simulink model "simulation"  (R2017b)
settings: Solver=VariableStepAuto  StartTime=0.0  StopTime=10.0  RelTol=1e-3
settings Model: Creator=max  LastModifiedBy=max

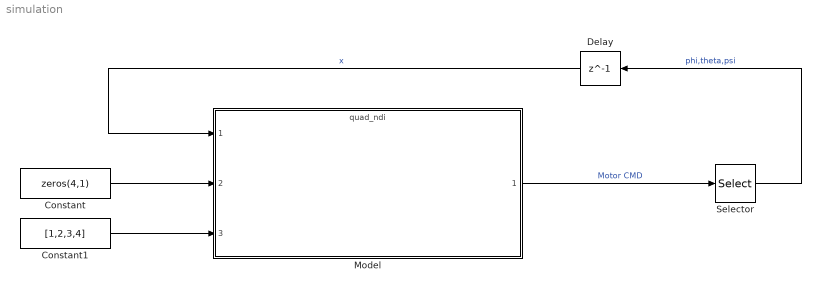
== system simulation ==
  Constant : Constant  Value=zeros(4,1)  OutDataTypeStr=single
  Constant1 : Constant  Value=[1,2,3,4]
  Delay : Delay  DelayLength=1  SampleTime=1/500
  Model : ModelReference  ModelNameDialog=quad_ndi.slx  SimulationMode=Normal  ModelReferenceVersion=1.585
  Selector : Selector  InputPortWidth=3  IndexOptions=Index vector (dialog)  Indices=[1 3]  OutputSizes=1
  wires:
  Model/1 -> Selector/1  "Motor CMD"
  Selector/1 -> Delay/1  "phi,theta,psi"
  Constant/1 -> Model/2
  Constant1/1 -> Model/3
  Delay/1 -> Model/1  "x"
